simulink model "Grua"  (R2024b)
settings: Solver=VariableStepAuto  StartTime=0.0  StopTime=35  RelTol=1e-3
values from neighbouring files (symbols this model uses):
  A = [0 0 0 0 0 0 0 -35.31 1 0 -9.431 0 ... (16 elements, 4x4)]    [GruaWorkspace.mat]    (also in grua.mat = [0 0 0 0 0 0 0 -35.3130710133 1 0 -9.69067245938 0 ... (16 e)
  A_a = [0 0 0 0 0 0 0 -74.151 2.1 0 -19.8051 0 ... (16 elements, 4x4)]    [GruaWorkspace.mat]
  AL = [0 0 0 0 0 0 0 -105.93 3 0 -28.293 0 ... (16 elements, 4x4)]    [GruaWorkspace.mat]
  B = [0 -0.2969 0.23092 -1.466]    [GruaWorkspace.mat]    (also in grua.mat = [0 -0.296894785399 0.236071876692 -1.46592019656])
  C1 = [1 0 0 0]    [GruaWorkspace.mat]    (also in grua.mat = [1  0  0  0; 0  1  0  0])
  K = [8.58461226427 -0.0859436500585 -6.5484588777 -2.00657807254]    [GruaWorkspace.mat]    (also in grua.mat = [11.2779924086 -1.98610202692 -5.28014178733 -2.15028681626])
  K1 = [11.2999971625 -2.14032234972 -4.67554747872 -2.14468343667]    [GruaWorkspace.mat]
  K_q = [46.2217629834 -33.8776196356 4.95214120639 -0.533590865229]    [GruaWorkspace.mat]    (also in grua.mat = [50.0170795212 -5.53286476625 6.72231103684 -0.384358946683])
  Ki = 2.83555961224    [GruaWorkspace.mat]    (also in grua.mat = 4.13832170273)
  Ki1 = 4.40025719588    [GruaWorkspace.mat]
  Ki_q = 17.6776695297    [GruaWorkspace.mat]    (also in grua.mat = 20)
libraries: simulink x3
settings Model: Creator=nagel  LastModifiedBy=wilbe

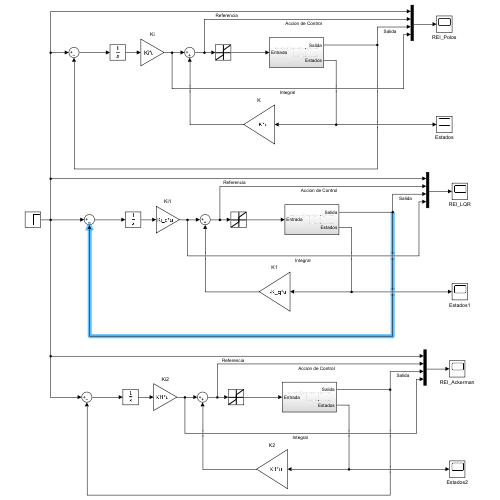
[thumbnail: Simulink's stored preview of the top-level diagram]
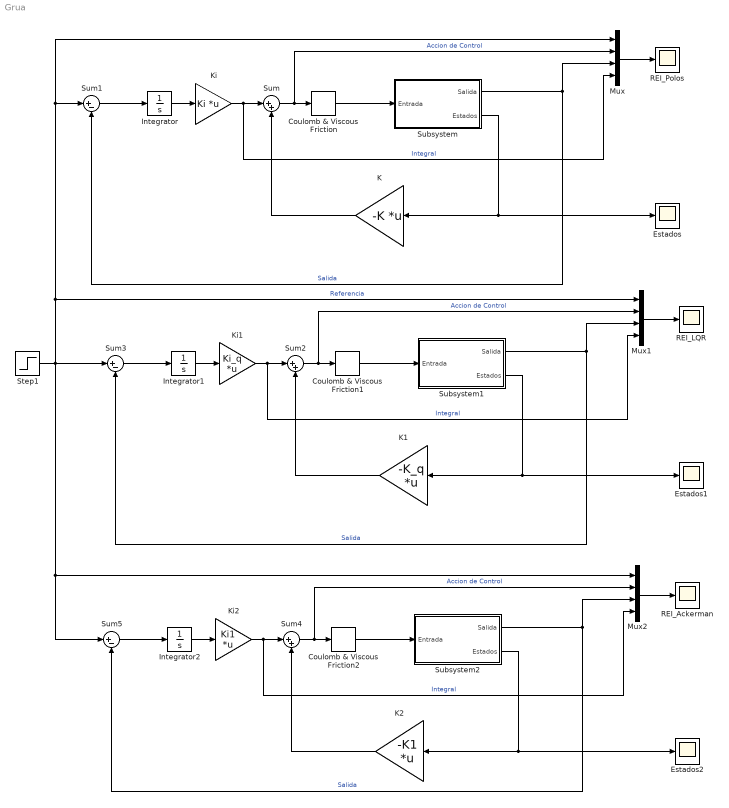
== system Grua ==
  Coulomb & Viscous Friction : simulink/Discontinuities/Coulomb & Viscous Friction  offset=[0.4]  gain=1
  Coulomb & Viscous Friction1 : simulink/Discontinuities/Coulomb & Viscous Friction  offset=[0.4]  gain=1
  Coulomb & Viscous Friction2 : simulink/Discontinuities/Coulomb & Viscous Friction  offset=[0.4]  gain=1
  Estados : Scope
  Estados1 : Scope
  Estados2 : Scope
  Integrator : Integrator
  Integrator1 : Integrator
  Integrator2 : Integrator
  K : Gain  Gain=-K  Multiplication=Matrix(K*u)
  K1 : Gain  Gain=-K_q  Multiplication=Matrix(K*u)
  K2 : Gain  Gain=-K1  Multiplication=Matrix(K*u)
  Ki : Gain  Gain=Ki  Multiplication=Matrix(K*u)
  Ki1 : Gain  Gain=Ki_q  Multiplication=Matrix(K*u)
  Ki2 : Gain  Gain=Ki1  Multiplication=Matrix(K*u)
  Mux : Mux
  Mux1 : Mux
  Mux2 : Mux
  REI_Ackerman : Scope
  REI_LQR : Scope
  REI_Polos : Scope
  Step1 : Step  Time=0  Before=1  SampleTime=0
  Subsystem : Subsystem
  Subsystem1 : Subsystem
  Subsystem2 : Subsystem
  Sum : Sum  Inputs=|++
  Sum1 : Sum  Inputs=|+-
  Sum2 : Sum  Inputs=|++
  Sum3 : Sum  Inputs=|+-
  Sum4 : Sum  Inputs=|++
  Sum5 : Sum  Inputs=|+-
  wires:
  Subsystem/1(Salida) -> Sum1/2, Mux/3  "Salida"
  Coulomb & Viscous Friction/1 -> Subsystem/1(Entrada)
  Subsystem/2(Estados) -> K/1, Estados/1
  Sum/1 -> Mux/2, Coulomb & Viscous Friction/1  "Accion de Control"
  K/1 -> Sum/2
  Integrator/1 -> Ki/1
  Ki/1 -> Mux/4, Sum/1  "Integral"
  Sum1/1 -> Integrator/1
  Mux/1 -> REI_Polos/1
  Step1/1 -> Mux1/1, Sum1/1, Mux/1, Sum3/1, Sum5/1, Mux2/1  "Referencia"
  Mux1/1 -> REI_LQR/1
  Subsystem1/1(Salida) -> Sum3/2, Mux1/3  "Salida"
  Sum3/1 -> Integrator1/1
  Integrator1/1 -> Ki1/1
  K1/1 -> Sum2/2
  Subsystem1/2(Estados) -> K1/1, Estados1/1
  Ki1/1 -> Mux1/4, Sum2/1  "Integral"
  Coulomb & Viscous Friction1/1 -> Subsystem1/1(Entrada)
  Sum2/1 -> Mux1/2, Coulomb & Viscous Friction1/1  "Accion de Control"
  Subsystem2/1(Salida) -> Sum5/2, Mux2/3  "Salida"
  Sum5/1 -> Integrator2/1
  Coulomb & Viscous Friction2/1 -> Subsystem2/1(Entrada)
  Ki2/1 -> Mux2/4, Sum4/1  "Integral"
  Sum4/1 -> Mux2/2, Coulomb & Viscous Friction2/1  "Accion de Control"
  Integrator2/1 -> Ki2/1
  Subsystem2/2(Estados) -> K2/1, Estados2/1
  K2/1 -> Sum4/2
  Mux2/1 -> REI_Ackerman/1

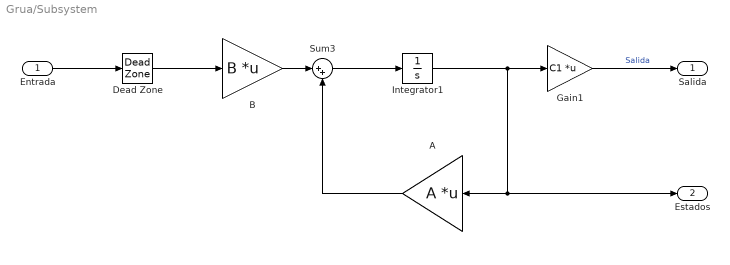
== system Grua/Subsystem ==
  Entrada : Inport
  A : Gain  Gain=A  Multiplication=Matrix(K*u)
  B : Gain  Gain=B  Multiplication=Matrix(K*u)
  Dead Zone : DeadZone  UpperValue=0.6
  Gain1 : Gain  Gain=C1  Multiplication=Matrix(K*u)
  Integrator1 : Integrator
  Sum3 : Sum  Inputs=|++
  Salida : Outport
  Estados : Outport  Port=2
  wires:
  Sum3/1 -> Integrator1/1
  B/1 -> Sum3/1
  A/1 -> Sum3/2
  Gain1/1 -> Salida/1  "Salida"
  Integrator1/1 -> A/1, Estados/1, Gain1/1
  Entrada/1 -> Dead Zone/1
  Dead Zone/1 -> B/1

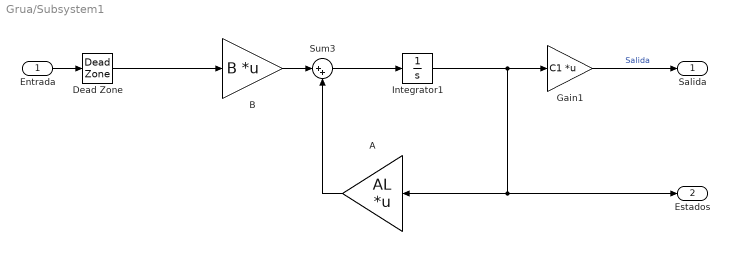
== system Grua/Subsystem1 ==
  Entrada : Inport
  A : Gain  Gain=AL  Multiplication=Matrix(K*u)
  B : Gain  Gain=B  Multiplication=Matrix(K*u)
  Dead Zone : DeadZone  UpperValue=0.6
  Gain1 : Gain  Gain=C1  Multiplication=Matrix(K*u)
  Integrator1 : Integrator
  Sum3 : Sum  Inputs=|++
  Salida : Outport
  Estados : Outport  Port=2
  wires:
  Sum3/1 -> Integrator1/1
  B/1 -> Sum3/1
  A/1 -> Sum3/2
  Gain1/1 -> Salida/1  "Salida"
  Integrator1/1 -> A/1, Estados/1, Gain1/1
  Entrada/1 -> Dead Zone/1
  Dead Zone/1 -> B/1

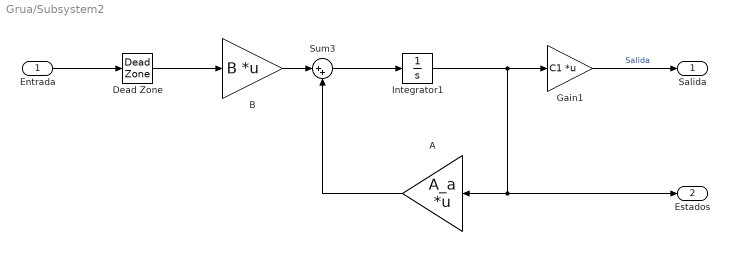
== system Grua/Subsystem2 ==
  Entrada : Inport
  A : Gain  Gain=A_a  Multiplication=Matrix(K*u)
  B : Gain  Gain=B  Multiplication=Matrix(K*u)
  Dead Zone : DeadZone  UpperValue=0.6
  Gain1 : Gain  Gain=C1  Multiplication=Matrix(K*u)
  Integrator1 : Integrator
  Sum3 : Sum  Inputs=|++
  Salida : Outport
  Estados : Outport  Port=2
  wires:
  Sum3/1 -> Integrator1/1
  B/1 -> Sum3/1
  A/1 -> Sum3/2
  Gain1/1 -> Salida/1  "Salida"
  Integrator1/1 -> A/1, Estados/1, Gain1/1
  Entrada/1 -> Dead Zone/1
  Dead Zone/1 -> B/1
